simulink model "reward"  (R2021b)
settings: Solver=VariableStepAuto  StartTime=0.0  StopTime=10.0  RelTol=1e-3
settings Model: Creator=mluser  LastModifiedBy=mluser

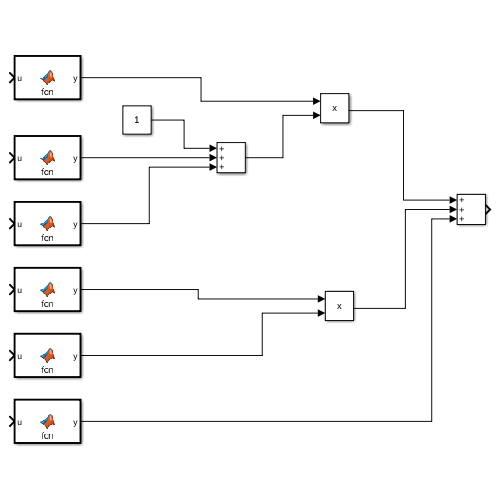
[thumbnail: Simulink's stored preview of the top-level diagram]
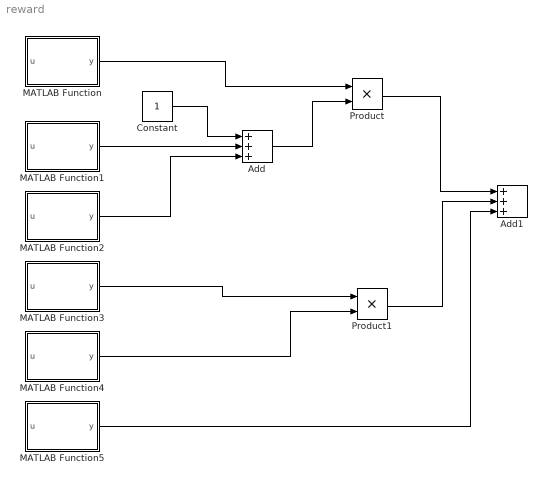
== system reward ==
  Add : Sum  Inputs=+++
  Add1 : Sum  Inputs=+++
  Constant : Constant
  MATLAB Function : MATLAB Function  TreatAsAtomicUnit=on
  MATLAB Function1 : MATLAB Function  TreatAsAtomicUnit=on
  MATLAB Function2 : MATLAB Function  TreatAsAtomicUnit=on
  MATLAB Function3 : MATLAB Function  TreatAsAtomicUnit=on
  MATLAB Function4 : MATLAB Function  TreatAsAtomicUnit=on
  MATLAB Function5 : MATLAB Function  TreatAsAtomicUnit=on
  Product : Product
  Product1 : Product
  wires:
  Constant/1 -> Add/1
  MATLAB Function1/1(y) -> Add/2
  MATLAB Function2/1(y) -> Add/3
  Add/1 -> Product/2
  MATLAB Function/1(y) -> Product/1
  MATLAB Function3/1(y) -> Product1/1
  MATLAB Function4/1(y) -> Product1/2
  Product/1 -> Add1/1
  Product1/1 -> Add1/2
  MATLAB Function5/1(y) -> Add1/3

== matlab function reward/MATLAB Function ==
  data: u input; y output
function y = fcn(u)

y = 2.0*exp(-0.5*(u^2)/0.1);

== matlab function reward/MATLAB Function2 ==
  data: u input; y output
function y = fcn(u)

y = 2.0*exp(-0.5*(u^2)/0.2);

== matlab function reward/MATLAB Function3 ==
  data: u input; y output
function y = fcn(u)

y = exp(-0.5*(u^2)/0.1);

== matlab function reward/MATLAB Function4 ==
  data: u input; y output
function y = fcn(u)
if abs(u) < 0.0164
    y = 0;
else 
    y = -30.6;
end

== matlab function reward/MATLAB Function5 ==
  data: u input; y output
function y = fcn(u)
if abs(u) < 0.25 
    y = 0;
else 
    y = -2.0;
end

== matlab function reward/MATLAB Function1 ==
  data: u input; y output
function y = fcn(u)

y = 0.5*exp(-0.5*(u^2)/0.005);
